simulink model "filter_ref"  (R2020b)
settings: Solver=VariableStepAuto  StartTime=0.0  StopTime=10.0  RelTol=1e-3
settings Model: Creator=Dell  LastModifiedBy=Dell
settings DataIOCC: SaveOutput=off  SaveTime=off

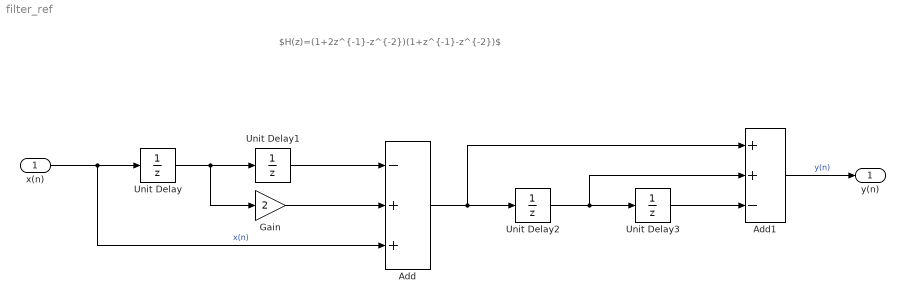
== system filter_ref ==
  note: $H(z)=(1+2z^{-1}-z^{-2})(1+z^{-1}-z^{-2})$
  x(n) : Inport  OutDataTypeStr=double  PortDimensions=1  SampleTime=[0,1]
  Add : Sum  Inputs=-++
  Add1 : Sum  Inputs=++-
  Gain : Gain  Gain=2
  Unit Delay{,1..3} (4 alike) : UnitDelay  SampleTime=-1  HasFrameUpgradeWarning=on
  y(n) : Outport  OutDataTypeStr=double  PortDimensions=1  SampleTime=[0,1]
  wires:
  Unit Delay2/1 -> Add1/2, Unit Delay3/1
  Gain/1 -> Add/2
  x(n)/1 -> Unit Delay/1, Add/3  "x(n)"
  Unit Delay1/1 -> Add/1
  Add1/1 -> y(n)/1  "y(n)"
  Unit Delay/1 -> Unit Delay1/1, Gain/1
  Add/1 -> Add1/1, Unit Delay2/1
  Unit Delay3/1 -> Add1/3
